simulink model "model"  (R2014a)
(part 6 of 6)

  L_188413965/LConn3 -- T_188413965__/RConn3 -- bus494/LConn1
  T_244288461_345000;230000;138000;88000;13800_Subestação_Anhangüera/RConn1 -- L_244288461/LConn1
  T_244288461_345000;230000;138000;88000;13800_Subestação_Anhangüera/RConn2 -- L_244288461/LConn2
  L_244288461/LConn3 -- T_244288461_345000;230000;138000;88000;13800_Subestação_Anhangüera/RConn3 -- bus495/LConn1
  T_152900437__/RConn1 -- L_152900437/LConn1
  T_152900437__/RConn2 -- L_152900437/LConn2
  L_152900437/LConn3 -- T_152900437__/RConn3 -- bus496/LConn1
  T_229464678__/RConn1 -- L_229464678/LConn1
  T_229464678__/RConn2 -- L_229464678/LConn2
  L_229464678/LConn3 -- T_229464678__/RConn3 -- bus497/LConn1
  T_189594688__/RConn1 -- L_189594688/LConn1
  T_189594688__/RConn2 -- L_189594688/LConn2
  L_189594688/LConn3 -- T_189594688__/RConn3 -- bus498/LConn1
  T_234150638__/RConn1 -- L_234150638/LConn1
  T_234150638__/RConn2 -- L_234150638/LConn2
  L_234150638/LConn3 -- T_234150638__/RConn3 -- bus499/LConn1
  T_169790429__Estação_elétrica/RConn1 -- L_169790429/LConn1
  T_169790429__Estação_elétrica/RConn2 -- L_169790429/LConn2
  L_169790429/LConn3 -- T_169790429__Estação_elétrica/RConn3 -- bus500/LConn1
  T_217382404__Usina_de_Jaguara/RConn1 -- L_217382404/LConn1
  T_217382404__Usina_de_Jaguara/RConn2 -- L_217382404/LConn2
  L_217382404/LConn3 -- T_217382404__Usina_de_Jaguara/RConn3 -- bus501/LConn1
  T_318426878__/RConn1 -- L_318426878/LConn1
  T_318426878__/RConn2 -- L_318426878/LConn2
  L_318426878/LConn3 -- T_318426878__/RConn3 -- bus502/LConn1
  T_226477359__/RConn1 -- L_226477359/LConn1
  T_226477359__/RConn2 -- L_226477359/LConn2
  L_226477359/LConn3 -- T_226477359__/RConn3 -- bus503/LConn1
  T_182621871__/RConn1 -- L_182621871/LConn1
  T_182621871__/RConn2 -- L_182621871/LConn2
  L_182621871/LConn3 -- T_182621871__/RConn3 -- bus504/LConn1
  T_132700720__/RConn1 -- L_132700720/LConn1
  T_132700720__/RConn2 -- L_132700720/LConn2
  L_132700720/LConn3 -- T_132700720__/RConn3 -- bus505/LConn1
  T_132700730__/RConn1 -- L_132700730/LConn1
  T_132700730__/RConn2 -- L_132700730/LConn2
  L_132700730/LConn3 -- T_132700730__/RConn3 -- bus506/LConn1
  T_175909703__/RConn1 -- L_175909703/LConn1
  T_175909703__/RConn2 -- L_175909703/LConn2
  L_175909703/LConn3 -- T_175909703__/RConn3 -- bus507/LConn1
  T_219471736__/RConn1 -- L_219471736/LConn1
  T_219471736__/RConn2 -- L_219471736/LConn2
  L_219471736/LConn3 -- T_219471736__/RConn3 -- bus508/LConn1
  T_132700759__/RConn1 -- L_132700759/LConn1
  T_132700759__/RConn2 -- L_132700759/LConn2
  L_132700759/LConn3 -- T_132700759__/RConn3 -- bus509/LConn1
  T_154269127__/RConn1 -- L_154269127/LConn1
  T_154269127__/RConn2 -- L_154269127/LConn2
  L_154269127/LConn3 -- T_154269127__/RConn3 -- bus510/LConn1
  T_174918846__/RConn1 -- L_174918846/LConn1
  T_174918846__/RConn2 -- L_174918846/LConn2
  L_174918846/LConn3 -- T_174918846__/RConn3 -- bus511/LConn1
  T_196782331__/RConn1 -- L_196782331/LConn1
  T_196782331__/RConn2 -- L_196782331/LConn2
  L_196782331/LConn3 -- T_196782331__/RConn3 -- bus512/LConn1
  T_319354712__/RConn1 -- L_319354712/LConn1
  T_319354712__/RConn2 -- L_319354712/LConn2
  L_319354712/LConn3 -- T_319354712__/RConn3 -- bus513/LConn1
  T_252205401__/RConn1 -- L_252205401/LConn1
  T_252205401__/RConn2 -- L_252205401/LConn2
  L_252205401/LConn3 -- T_252205401__/RConn3 -- bus514/LConn1
  T_197950082__/RConn1 -- L_197950082/LConn1
  T_197950082__/RConn2 -- L_197950082/LConn2
  L_197950082/LConn3 -- T_197950082__/RConn3 -- bus515/LConn1
  T_172071437__/RConn1 -- L_172071437/LConn1
  T_172071437__/RConn2 -- L_172071437/LConn2
  L_172071437/LConn3 -- T_172071437__/RConn3 -- bus516/LConn1
  T_160888682__/RConn1 -- L_160888682/LConn1
  T_160888682__/RConn2 -- L_160888682/LConn2
  L_160888682/LConn3 -- T_160888682__/RConn3 -- bus517/LConn1
  T_175929233__Subestação_de_Santo_Ângelo/RConn1 -- L_175929233/LConn1
  T_175929233__Subestação_de_Santo_Ângelo/RConn2 -- L_175929233/LConn2
  L_175929233/LConn3 -- T_175929233__Subestação_de_Santo_Ângelo/RConn3 -- bus518/LConn1
  T_218090562__Subestação_de_Energia_Elétrica_Cteep/RConn1 -- L_218090562/LConn1
  T_218090562__Subestação_de_Energia_Elétrica_Cteep/RConn2 -- L_218090562/LConn2
  L_218090562/LConn3 -- T_218090562__Subestação_de_Energia_Elétrica_Cteep/RConn3 -- bus519/LConn1
  T_171525061__Subestação/RConn1 -- L_171525061/LConn1
  T_171525061__Subestação/RConn2 -- L_171525061/LConn2
  L_171525061/LConn3 -- T_171525061__Subestação/RConn3 -- bus520/LConn1
  T_244245455__/RConn1 -- L_244245455/LConn1
  T_244245455__/RConn2 -- L_244245455/LConn2
  L_244245455/LConn3 -- T_244245455__/RConn3 -- bus521/LConn1
  T_341042754__CESP/RConn1 -- L_341042754/LConn1
  T_341042754__CESP/RConn2 -- L_341042754/LConn2
  L_341042754/LConn3 -- T_341042754__CESP/RConn3 -- bus522/LConn1
  T_183163485__/RConn1 -- L_183163485/LConn1
  T_183163485__/RConn2 -- L_183163485/LConn2
  L_183163485/LConn3 -- T_183163485__/RConn3 -- bus523/LConn1
  T_167339557__/RConn1 -- L_167339557/LConn1
  T_167339557__/RConn2 -- L_167339557/LConn2
  L_167339557/LConn3 -- T_167339557__/RConn3 -- bus524/LConn1
  T_286006777_440000_/RConn1 -- L_286006777/LConn1
  T_286006777_440000_/RConn2 -- L_286006777/LConn2
  L_286006777/LConn3 -- T_286006777_440000_/RConn3 -- bus525/LConn1
  T_172691560__/RConn1 -- L_172691560/LConn1
  T_172691560__/RConn2 -- L_172691560/LConn2
  L_172691560/LConn3 -- T_172691560__/RConn3 -- bus526/LConn1
  T_156042539__/RConn1 -- L_156042539/LConn1
  T_156042539__/RConn2 -- L_156042539/LConn2
  L_156042539/LConn3 -- T_156042539__/RConn3 -- bus527/LConn1
  T_296110000__/RConn1 -- L_296110000/LConn1
  T_296110000__/RConn2 -- L_296110000/LConn2
  L_296110000/LConn3 -- T_296110000__/RConn3 -- bus528/LConn1
  T_286007002_440000_/RConn1 -- L_286007002/LConn1
  T_286007002_440000_/RConn2 -- L_286007002/LConn2
  L_286007002/LConn3 -- T_286007002_440000_/RConn3 -- bus529/LConn1
  T_302735025_440000_/RConn1 -- L_302735025/LConn1
  T_302735025_440000_/RConn2 -- L_302735025/LConn2
  L_302735025/LConn3 -- T_302735025_440000_/RConn3 -- bus530/LConn1
  T_302901044__/RConn1 -- L_302901044/LConn1
  T_302901044__/RConn2 -- L_302901044/LConn2
  L_302901044/LConn3 -- T_302901044__/RConn3 -- bus531/LConn1
  T_174017677_440000_/RConn1 -- L_174017677/LConn1
  T_174017677_440000_/RConn2 -- L_174017677/LConn2
  L_174017677/LConn3 -- T_174017677_440000_/RConn3 -- bus532/LConn1
  T_186982606__/RConn1 -- L_186982606/LConn1
  T_186982606__/RConn2 -- L_186982606/LConn2
  L_186982606/LConn3 -- T_186982606__/RConn3 -- bus533/LConn1
  T_323557393__/RConn1 -- L_323557393/LConn1
  T_323557393__/RConn2 -- L_323557393/LConn2
  L_323557393/LConn3 -- T_323557393__/RConn3 -- bus534/LConn1
  T_271191830__Subestação_Colinas/RConn1 -- L_271191830/LConn1
  T_271191830__Subestação_Colinas/RConn2 -- L_271191830/LConn2
  L_271191830/LConn3 -- T_271191830__Subestação_Colinas/RConn3 -- bus535/LConn1
  T_304139576__/RConn1 -- L_304139576/LConn1
  T_304139576__/RConn2 -- L_304139576/LConn2
  L_304139576/LConn3 -- T_304139576__/RConn3 -- bus536/LConn1
  T_249499770__/RConn1 -- L_249499770/LConn1
  T_249499770__/RConn2 -- L_249499770/LConn2
  L_249499770/LConn3 -- T_249499770__/RConn3 -- bus537/LConn1
  T_271524307__Subestação_da_Eletronorte_em_Marabá/RConn1 -- L_271524307/LConn1
  T_271524307__Subestação_da_Eletronorte_em_Marabá/RConn2 -- L_271524307/LConn2
  L_271524307/LConn3 -- T_271524307__Subestação_da_Eletronorte_em_Marabá/RConn3 -- bus538/LConn1
  T_176499706__Açailândia/RConn1 -- L_176499706/LConn1
  T_176499706__Açailândia/RConn2 -- L_176499706/LConn2
  L_176499706/LConn3 -- T_176499706__Açailândia/RConn3 -- bus539/LConn1
  T_262913646__/RConn1 -- L_262913646/LConn1
  T_262913646__/RConn2 -- L_262913646/LConn2
  L_262913646/LConn3 -- T_262913646__/RConn3 -- bus540/LConn1
  T_171525050__/RConn1 -- L_171525050/LConn1
  T_171525050__/RConn2 -- L_171525050/LConn2
  L_171525050/LConn3 -- T_171525050__/RConn3 -- bus541/LConn1
  T_167516187__Subestação_Batéias/RConn1 -- L_167516187/LConn1
  T_167516187__Subestação_Batéias/RConn2 -- L_167516187/LConn2
  L_167516187/LConn3 -- T_167516187__Subestação_Batéias/RConn3 -- bus542/LConn1
  T_154030807__/RConn1 -- L_154030807/LConn1
  T_154030807__/RConn2 -- L_154030807/LConn2
  L_154030807/LConn3 -- T_154030807__/RConn3 -- bus543/LConn1
  T_229733923__Subestação_Rio_Verde_Norte/RConn1 -- L_229733923/LConn1
  T_229733923__Subestação_Rio_Verde_Norte/RConn2 -- L_229733923/LConn2
  L_229733923/LConn3 -- T_229733923__Subestação_Rio_Verde_Norte/RConn3 -- bus544/LConn1
  T_228748856__Gravataí/RConn1 -- L_228748856/LConn1
  T_228748856__Gravataí/RConn2 -- L_228748856/LConn2
  L_228748856/LConn3 -- T_228748856__Gravataí/RConn3 -- bus545/LConn1
  T_247684836__/RConn1 -- L_247684836/LConn1
  T_247684836__/RConn2 -- L_247684836/LConn2
  L_247684836/LConn3 -- T_247684836__/RConn3 -- bus546/LConn1
  T_252169283__Subestação_Vespasiano_2/RConn1 -- L_252169283/LConn1
  T_252169283__Subestação_Vespasiano_2/RConn2 -- L_252169283/LConn2
  L_252169283/LConn3 -- T_252169283__Subestação_Vespasiano_2/RConn3 -- bus547/LConn1
  T_252169286__Subestação_Neves_1/RConn1 -- L_252169286/LConn1
  T_252169286__Subestação_Neves_1/RConn2 -- L_252169286/LConn2
  L_252169286/LConn3 -- T_252169286__Subestação_Neves_1/RConn3 -- bus548/LConn1
  T_297523069__Sub_Estação_da_CEMIG___Bom_Despacho/RConn1 -- L_297523069/LConn1
  T_297523069__Sub_Estação_da_CEMIG___Bom_Despacho/RConn2 -- L_297523069/LConn2
  L_297523069/LConn3 -- T_297523069__Sub_Estação_da_CEMIG___Bom_Despacho/RConn3 -- bus549/LConn1
  T_253440615__/RConn1 -- L_253440615/LConn1
  T_253440615__/RConn2 -- L_253440615/LConn2
  L_253440615/LConn3 -- T_253440615__/RConn3 -- bus550/LConn1
  T_253030804__Serra_da_Mesa/RConn1 -- L_253030804/LConn1
  T_253030804__Serra_da_Mesa/RConn2 -- L_253030804/LConn2
  L_253030804/LConn3 -- T_253030804__Serra_da_Mesa/RConn3 -- bus551/LConn1
  T_253441434__/RConn1 -- L_253441434/LConn1
  T_253441434__/RConn2 -- L_253441434/LConn2
  L_253441434/LConn3 -- T_253441434__/RConn3 -- bus552/LConn1
  T_253692682__/RConn1 -- L_253692682/LConn1
  T_253692682__/RConn2 -- L_253692682/LConn2
  L_253692682/LConn3 -- T_253692682__/RConn3 -- bus553/LConn1
  T_262559849__/RConn1 -- L_262559849/LConn1
  T_262559849__/RConn2 -- L_262559849/LConn2
  L_262559849/LConn3 -- T_262559849__/RConn3 -- bus554/LConn1
  T_244422281__Paracatu_4/RConn1 -- L_244422281/LConn1
  T_244422281__Paracatu_4/RConn2 -- L_244422281/LConn2
  L_244422281/LConn3 -- T_244422281__Paracatu_4/RConn3 -- bus555/LConn1
  T_158099916__Pirapora_2/RConn1 -- L_158099916/LConn1
  T_158099916__Pirapora_2/RConn2 -- L_158099916/LConn2
  L_158099916/LConn3 -- T_158099916__Pirapora_2/RConn3 -- bus556/LConn1
  T_283488616__Subestação_de_Emborcação/RConn1 -- L_283488616/LConn1
  T_283488616__Subestação_de_Emborcação/RConn2 -- L_283488616/LConn2
  L_283488616/LConn3 -- T_283488616__Subestação_de_Emborcação/RConn3 -- bus557/LConn1
  T_259229502__/RConn1 -- L_259229502/LConn1
  T_259229502__/RConn2 -- L_259229502/LConn2
  L_259229502/LConn3 -- T_259229502__/RConn3 -- bus558/LConn1
  T_259425260__/RConn1 -- L_259425260/LConn1
  T_259425260__/RConn2 -- L_259425260/LConn2
  L_259425260/LConn3 -- T_259425260__/RConn3 -- bus559/LConn1
  T_320600714__Subestação_Rio_das_Éguas/RConn1 -- L_320600714/LConn1
  T_320600714__Subestação_Rio_das_Éguas/RConn2 -- L_320600714/LConn2
  L_320600714/LConn3 -- T_320600714__Subestação_Rio_das_Éguas/RConn3 -- bus560/LConn1
  T_188465343__/RConn1 -- L_188465343/LConn1
  T_188465343__/RConn2 -- L_188465343/LConn2
  L_188465343/LConn3 -- T_188465343__/RConn3 -- bus561/LConn1
  T_204484095__/RConn1 -- L_204484095/LConn1
  T_204484095__/RConn2 -- L_204484095/LConn2
  L_204484095/LConn3 -- T_204484095__/RConn3 -- bus562/LConn1
  T_142588064__Hidroelétrica_de_Sobradinho/RConn1 -- L_142588064/LConn1
  T_142588064__Hidroelétrica_de_Sobradinho/RConn2 -- L_142588064/LConn2
  L_142588064/LConn3 -- T_142588064__Hidroelétrica_de_Sobradinho/RConn3 -- bus563/LConn1
  T_390650768__/RConn1 -- L_390650768/LConn1
  T_390650768__/RConn2 -- L_390650768/LConn2
  L_390650768/LConn3 -- T_390650768__/RConn3 -- bus564/LConn1
  T_150728359__Subestação_Segredo/RConn1 -- L_150728359/LConn1
  T_150728359__Subestação_Segredo/RConn2 -- L_150728359/LConn2
  L_150728359/LConn3 -- T_150728359__Subestação_Segredo/RConn3 -- bus565/LConn1
  T_150728360__/RConn1 -- L_150728360/LConn1
  T_150728360__/RConn2 -- L_150728360/LConn2
  L_150728360/LConn3 -- T_150728360__/RConn3 -- bus566/LConn1
  T_125761911__/RConn1 -- L_125761911/LConn1
  T_125761911__/RConn2 -- L_125761911/LConn2
  L_125761911/LConn3 -- T_125761911__/RConn3 -- bus567/LConn1
  T_204662229__/RConn1 -- L_204662229/LConn1
  T_204662229__/RConn2 -- L_204662229/LConn2
  L_204662229/LConn3 -- T_204662229__/RConn3 -- bus568/LConn1
  T_253523129__Subestação_UHE_Serra_da_Mesa/RConn1 -- L_253523129/LConn1
  T_253523129__Subestação_UHE_Serra_da_Mesa/RConn2 -- L_253523129/LConn2
  L_253523129/LConn3 -- T_253523129__Subestação_UHE_Serra_da_Mesa/RConn3 -- bus569/LConn1
  T_32302779__/RConn1 -- L_32302779/LConn1
  T_32302779__/RConn2 -- L_32302779/LConn2
  L_32302779/LConn3 -- T_32302779__/RConn3 -- bus570/LConn1
  T_216693990__/RConn1 -- L_216693990/LConn1
  T_216693990__/RConn2 -- L_216693990/LConn2
  L_216693990/LConn3 -- T_216693990__/RConn3 -- bus571/LConn1
  T_174906606__/RConn1 -- L_174906606/LConn1
  T_174906606__/RConn2 -- L_174906606/LConn2
  L_174906606/LConn3 -- T_174906606__/RConn3 -- bus572/LConn1
  T_198634993__/RConn1 -- L_198634993/LConn1
  T_198634993__/RConn2 -- L_198634993/LConn2
  L_198634993/LConn3 -- T_198634993__/RConn3 -- bus573/LConn1
  T_280057613__Subestação_de_Xingó___CHESF/RConn1 -- L_280057613/LConn1
  T_280057613__Subestação_de_Xingó___CHESF/RConn2 -- L_280057613/LConn2
  L_280057613/LConn3 -- T_280057613__Subestação_de_Xingó___CHESF/RConn3 -- bus574/LConn1
  T_247537019__Subestação_CROP/RConn1 -- L_247537019/LConn1
  T_247537019__Subestação_CROP/RConn2 -- L_247537019/LConn2
  L_247537019/LConn3 -- T_247537019__Subestação_CROP/RConn3 -- bus575/LConn1
  T_304658726__/RConn1 -- L_304658726/LConn1
  T_304658726__/RConn2 -- L_304658726/LConn2
  L_304658726/LConn3 -- T_304658726__/RConn3 -- bus576/LConn1
  T_129484075__Subestação_de_Furnas/RConn1 -- L_129484075/LConn1
  T_129484075__Subestação_de_Furnas/RConn2 -- L_129484075/LConn2
  L_129484075/LConn3 -- T_129484075__Subestação_de_Furnas/RConn3 -- bus577/LConn1
  T_380022067__/RConn1 -- L_380022067/LConn1
  T_380022067__/RConn2 -- L_380022067/LConn2
  L_380022067/LConn3 -- T_380022067__/RConn3 -- bus578/LConn1
  T_202622375__/RConn1 -- L_202622375/LConn1
  T_202622375__/RConn2 -- L_202622375/LConn2
  L_202622375/LConn3 -- T_202622375__/RConn3 -- bus579/LConn1
